simulink model "LabSim"  (R2020b)
settings: Solver=ode4  StartTime=0.0  StopTime=100  FixedStep=0.001  RelTol=1e-3
values from neighbouring files (symbols this model uses):
  alphaInt = 6*pi/180    (= 0.10471975512)    [FindingNets.m]
  c = 0.0012    [DataGen.m]    (also in FindingNets.m)
  f = 0.000136    [DataGen.m]    (also in FindingNets.m)
  g = 9.798    [DataGen.m]    (also in FindingNets.m)
  Ipend = (Mwheel+Mmotor+Mrod/4)*l^2+Iextra    (= 0.02444648066)    [DataGen.m]    (also in FindingNets.m = 0.02434648066)
  Jtot = Jwheel+Jmotor    (= 0.00064925)    [DataGen.m]    (also in FindingNets.m)
  ke = 60/(2*pi*374)/2    (= 0.0127664392854)    [DataGen.m]    (also in FindingNets.m)
  kt = (25.5e-3)/2    (= 0.01275)    [DataGen.m]    (also in FindingNets.m)
  l = 0.2566    [DataGen.m]    (also in FindingNets.m)
  Mpend = Mwheel+Mmotor+Mrod/2    (= 0.381)    [DataGen.m]    (also in FindingNets.m)
  R = 1.2    [DataGen.m]    (also in FindingNets.m)
  StopTime = 5    [DataGen.m]    (also in FindingNets.m = 10)
  W1 = double(net.Layers(3).Weights)    [FindingNets.m]
  W1_b = double(net.Layers(3).Bias)    [FindingNets.m]
  W2 = double(net.Layers(5).Weights)    [FindingNets.m]
  W2_b = double(net.Layers(5).Bias)    [FindingNets.m]
  W3 = double(net.Layers(7).Weights)    [FindingNets.m]
  W3_b = double(net.Layers(7).Bias)    [FindingNets.m]
libraries: simulink x1
settings Model: Creator=Tzahi  LastModifiedBy=yizhak

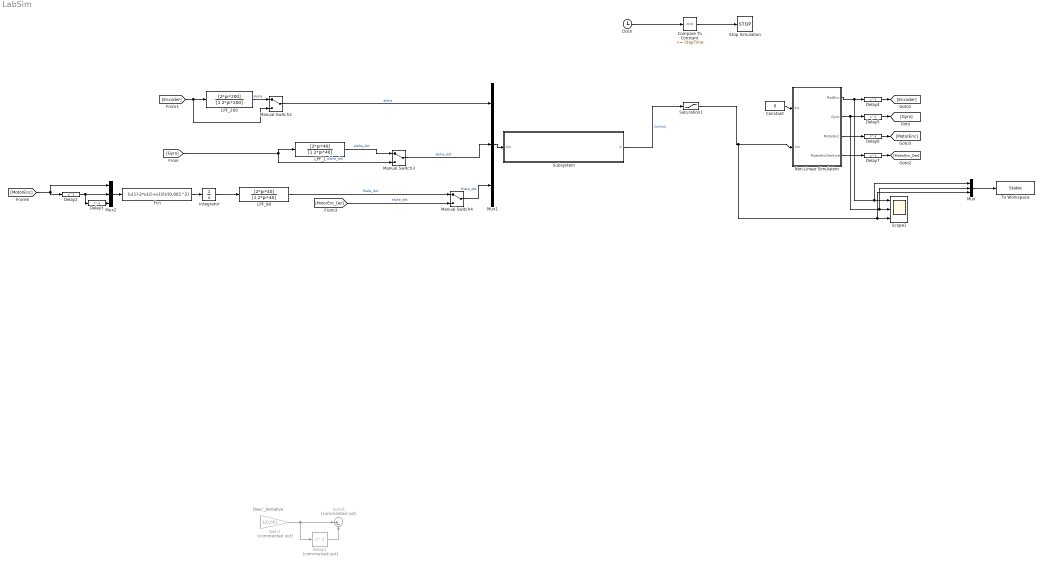
== system LabSim ==
  note: Desc'_deriative
  Clock : Clock
  Compare To Constant : simulink/Logic and Bit Operations/Compare To Constant  relop=>=  const=StopTime  OutDataTypeStr=boolean
  Constant : Constant  Value=0
  Delay1 : Delay  Commented=on  DelayLength=1
  Delay{2..7} (6 alike) : Delay  DelayLength=1
  Fcn : Fcn  Expr=(u(1)-2*u(2)+u(3))/(0.001^2)
  Gain7 : Gain  Commented=on  Gain=1/0.001
  Integrator : Integrator
  LPF_1 : TransferFcn  Numerator=[2*pi*40]  Denominator=[1 2*pi*40]
  LPF_200 : TransferFcn  Numerator=[2*pi*200]  Denominator=[1 2*pi*200]
  LPF_80 : TransferFcn  Numerator=[2*pi*40]  Denominator=[1 2*pi*40]
  Manual Switch2 : ManualSwitch
  Manual Switch3 : ManualSwitch
  Manual Switch4 : ManualSwitch
  Mux : Mux  Inputs=3
  Mux1 : Mux  Inputs=3
  Mux2 : Mux  Inputs=3
  Non-Linear Simulation : Subsystem
  Saturation1 : Saturate  UpperLimit=12  LowerLimit=-12
  Scope1 : Scope  NumInputPorts=3
  Stop Simulation : Stop
  Subsystem : Subsystem
  Sum6 : Sum  Commented=on  Inputs=|+-
  To Workspace : ToWorkspace  VariableName=States  SaveFormat=Timeseries  SampleTime=-1
  wires:
  [MotorEnc] -> Mux2/1, Delay2/1
  Delay1/1 -> Sum6/2
  Gain7/1 -> Delay1/1, Sum6/1
  Subsystem/1(V) -> Saturation1/1  "Control"
  Manual Switch4/1 -> Mux1/3  "theta_dot"
  Fcn/1 -> Integrator/1
  Mux1/1 -> Subsystem/1(Xin)
  Manual Switch2/1 -> Mux1/1  "alpha"
  Manual Switch3/1 -> Mux1/2  "alpha_dot"
  [Encoder] -> Manual Switch2/2, LPF_200/1
  Constant/1 -> Non-Linear Simulation/1(Td)
  Non-Linear Simulation/1(RodEnc) -> Delay4/1, Mux/1, Scope1/1
  Non-Linear Simulation/2(Gyro) -> Mux/2, Scope1/2, Delay5/1
  Non-Linear Simulation/3(MotorEnc) -> Delay6/1
  [Gyro] -> LPF_1/1, Manual Switch3/2  "alpha_dot"
  Compare To Constant/1 -> Stop Simulation/1
  Clock/1 -> Compare To Constant/1
  Mux/1 -> To Workspace/1
  LPF_200/1 -> Manual Switch2/1  "alpha"
  LPF_1/1 -> Manual Switch3/1  "alpha_dot"
  LPF_80/1 -> Manual Switch4/1  "theta_dot"
  Saturation1/1 -> Non-Linear Simulation/2(Vin), Mux/3, Scope1/3
  Non-Linear Simulation/4(MotorEncDeritive) -> Delay7/1
  [MotorEnc_Der] -> Manual Switch4/2  "alpha_dot"
  Integrator/1 -> LPF_80/1
  Mux2/1 -> Fcn/1
  Delay2/1 -> Delay3/1, Mux2/2
  Delay3/1 -> Mux2/3
  Delay5/1 -> [Gyro]
  Delay6/1 -> [MotorEnc]
  Delay7/1 -> [MotorEnc_Der]
  Delay4/1 -> [Encoder]

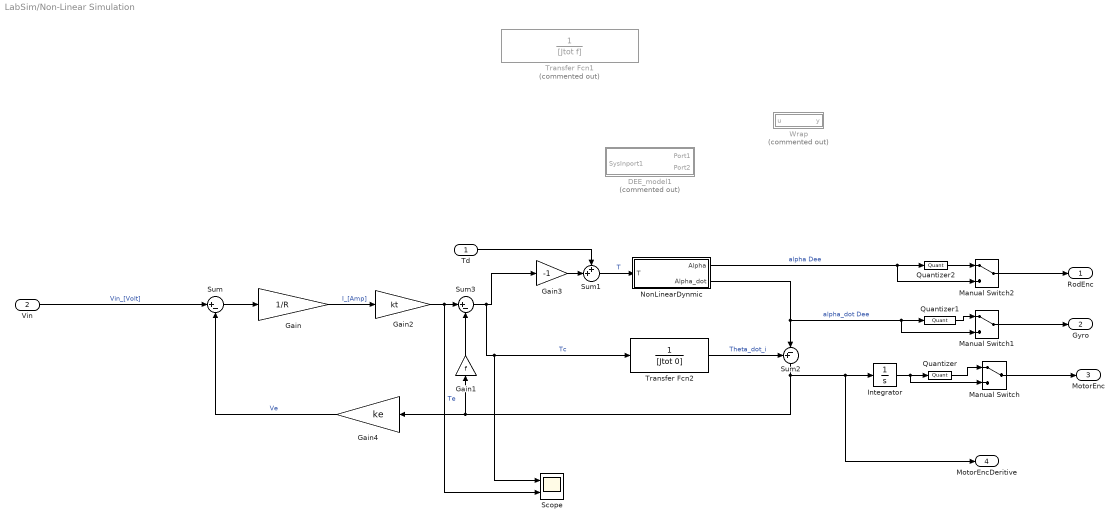
== system LabSim/Non-Linear Simulation ==
  Td : Inport
  Vin : Inport  Port=2
  DEE_model1 : Subsystem  Commented=on  mask(Differential Equation Editor (DEE)){}
      settings: OpenFcn=diffeqed
      mask Display: disp('pendalium')
  Gain : Gain  Gain=1/R
  Gain1 : Gain  Gain=f
  Gain2 : Gain  Gain=kt
  Gain3 : Gain  Gain=-1
  Gain4 : Gain  Gain=ke
  Integrator : Integrator
  Manual Switch : ManualSwitch
  Manual Switch1 : ManualSwitch
  Manual Switch2 : ManualSwitch
  NonLinearDynmic : Subsystem
  Quantizer : Quantizer  QuantizationInterval=(2*pi)/32
  Quantizer1 : Quantizer  QuantizationInterval=0.018
  Quantizer2 : Quantizer  QuantizationInterval=2*pi/500
  Scope : Scope  NumInputPorts=2
  Sum : Sum  Inputs=|+-
  Sum1 : Sum  Inputs=++|
  Sum2 : Sum  Inputs=+-|
  Sum3 : Sum  Inputs=|+-
  Transfer Fcn1 : TransferFcn  Commented=on  Denominator=[Jtot f]
  Transfer Fcn2 : TransferFcn  Denominator=[Jtot 0]
  Wrap : MATLAB Function  Commented=on  TreatAsAtomicUnit=on
  RodEnc : Outport
  Gyro : Outport  Port=2
  MotorEnc : Outport  Port=3
  MotorEncDeritive : Outport  Port=4
  wires:
  Sum2/1 -> MotorEncDeritive/1, Integrator/1, Gain4/1, Gain1/1
  Quantizer/1 -> Manual Switch/1
  Integrator/1 -> Manual Switch/2, Quantizer/1
  Quantizer1/1 -> Manual Switch1/1
  Gain1/1 -> Sum3/2
  Gain2/1 -> Scope/2, Sum3/1  "Te"
  Sum/1 -> Gain/1
  NonLinearDynmic/1(Alpha) -> Manual Switch2/2, Quantizer2/1  "alpha Dee"
  NonLinearDynmic/2(Alpha_dot) -> Sum2/2, Manual Switch1/2, Quantizer1/1  "alpha_dot Dee"
  Td/1 -> Sum1/1
  Sum1/1 -> NonLinearDynmic/1(T)  "T"
  Gain4/1 -> Sum/2  "Ve"
  Vin/1 -> Sum/1  "Vin_[Volt]"
  Sum3/1 -> Gain3/1, Scope/1, Transfer Fcn2/1  "Tc"
  Transfer Fcn2/1 -> Sum2/1  "Theta_dot_i"
  Gain3/1 -> Sum1/2
  Gain/1 -> Gain2/1  "I_[Amp]"
  Quantizer2/1 -> Manual Switch2/1
  Manual Switch/1 -> MotorEnc/1
  Manual Switch1/1 -> Gyro/1
  Manual Switch2/1 -> RodEnc/1

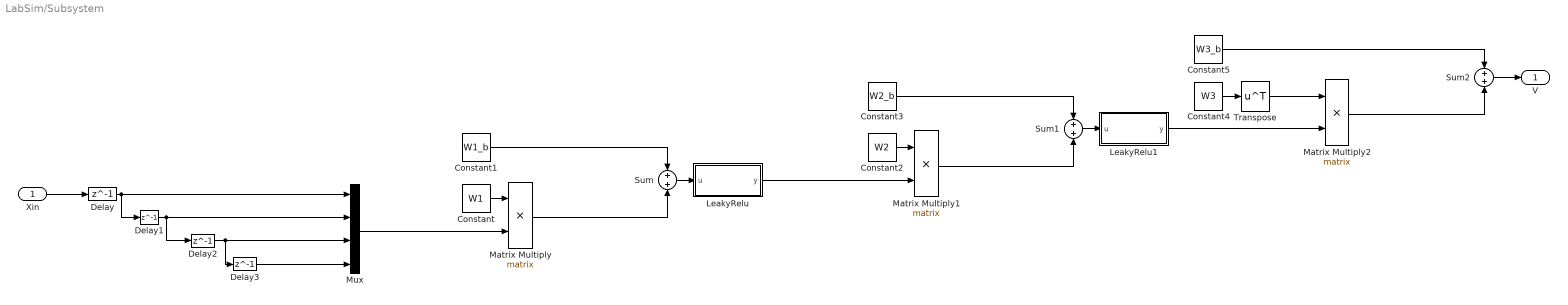
== system LabSim/Subsystem ==
  Xin : Inport
  Constant : Constant  Value=W1
  Constant1 : Constant  Value=W1_b
  Constant2 : Constant  Value=W2
  Constant3 : Constant  Value=W2_b
  Constant4 : Constant  Value=W3
  Constant5 : Constant  Value=W3_b
  Delay{,1..3} (4 alike) : Delay  DelayLength=1
  LeakyRelu : MATLAB Function  TreatAsAtomicUnit=on
  LeakyRelu1 : MATLAB Function  TreatAsAtomicUnit=on
  Matrix Multiply : Product  Multiplication=Matrix(*)
  Matrix Multiply1 : Product  Multiplication=Matrix(*)
  Matrix Multiply2 : Product  Multiplication=Matrix(*)
  Mux : Mux
  Sum : Sum
  Sum1 : Sum
  Sum2 : Sum
  Transpose : Math  Operator=transpose  SignedPower=on  SaturateOnIntegerOverflow=on
  V : Outport  VectorParamsAs1DForOutWhenUnconnected=off
  wires:
  Transpose/1 -> Matrix Multiply2/1
  Sum2/1 -> V/1
  Constant5/1 -> Sum2/1
  Matrix Multiply2/1 -> Sum2/2
  Constant4/1 -> Transpose/1
  LeakyRelu1/1(y) -> Matrix Multiply2/2
  LeakyRelu/1(y) -> Matrix Multiply1/2
  Constant2/1 -> Matrix Multiply1/1
  Matrix Multiply1/1 -> Sum1/2
  Constant3/1 -> Sum1/1
  Sum1/1 -> LeakyRelu1/1(u)
  Sum/1 -> LeakyRelu/1(u)
  Constant1/1 -> Sum/1
  Matrix Multiply/1 -> Sum/2
  Constant/1 -> Matrix Multiply/1
  Delay/1 -> Mux/1, Delay1/1
  Delay3/1 -> Mux/4
  Delay1/1 -> Mux/2, Delay2/1
  Xin/1 -> Delay/1
  Delay2/1 -> Mux/3, Delay3/1
  Mux/1 -> Matrix Multiply/2

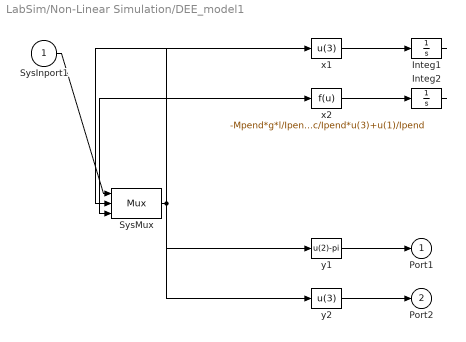
== system LabSim/Non-Linear Simulation/DEE_model1 ==
  SysInport1 : Inport
  Integ1 : Integrator  InitialCondition=+pi+alphaInt
  Integ2 : Integrator
  SysMux : Mux  Inputs=3
  x1 : Fcn  Expr=u(3)
  x2 : Fcn  Expr=-Mpend*g*l/Ipend*sin(u(2)) -c/Ipend*u(3)+u(1)/Ipend
  y1 : Fcn  Expr=u(2)-pi
  y2 : Fcn  Expr=u(3)
  Port1 : Outport  InitialOutput=0
  Port2 : Outport  Port=2  InitialOutput=0
  wires:
  y2/1 -> Port2/1
  y1/1 -> Port1/1
  Integ2/1 -> SysMux/3
  x2/1 -> Integ2/1
  Integ1/1 -> SysMux/2
  x1/1 -> Integ1/1
  SysMux/1 -> y2/1, y1/1, x2/1, x1/1
  SysInport1/1 -> SysMux/1

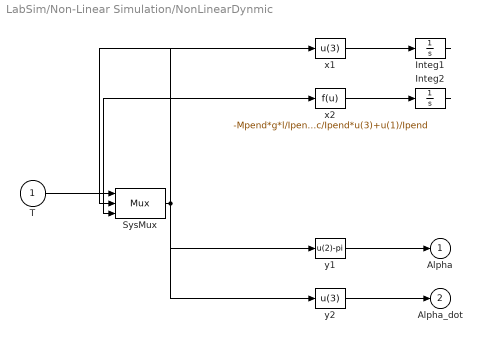
== system LabSim/Non-Linear Simulation/NonLinearDynmic ==
  T : Inport
  Integ1 : Integrator  InitialCondition=+pi+alphaInt
  Integ2 : Integrator
  SysMux : Mux  Inputs=3
  x1 : Fcn  Expr=u(3)
  x2 : Fcn  Expr=-Mpend*g*l/Ipend*sin(u(2)) -c/Ipend*u(3)+u(1)/Ipend
  y1 : Fcn  Expr=u(2)-pi
  y2 : Fcn  Expr=u(3)
  Alpha : Outport  InitialOutput=0
  Alpha_dot : Outport  Port=2  InitialOutput=0
  wires:
  T/1 -> SysMux/1
  x1/1 -> Integ1/1
  y2/1 -> Alpha_dot/1
  x2/1 -> Integ2/1
  Integ2/1 -> SysMux/3
  y1/1 -> Alpha/1
  SysMux/1 -> x1/1, x2/1, y1/1, y2/1
  Integ1/1 -> SysMux/2

== matlab function LabSim/Subsystem/LeakyRelu1 ==
  data: u input; y output
function y = fcn(u)
u(find(u<0))=0.4*u(find(u<0));
y = u;

== matlab function LabSim/Non-Linear Simulation/Wrap ==
  data: u input; y output
function y = Warp_pi(u)

y = atan2(sin(u),cos(u));

== matlab function LabSim/Subsystem/LeakyRelu ==
  data: u input; y output
function y = fcn(u)
u(find(u<0))=0.5*u(find(u<0));
y = u;
